simulink model "optical_path"  (R2016a)
settings: Solver=FixedStepDiscrete  StartTime=0.0  StopTime=250  FixedStep=0.1  RelTol=1e-3
undefined symbols (not defined in the file or in its folder): K, R
libraries: CEO x3
settings Model: Creator=rconan  LastModifiedBy=rconan
settings DataIOCC: LimitDataPoints=on  SaveFormat=Array
settings HardwareCC: ProdBitPerPointer=32  ProdLargestAtomicFloat=None  ProdIntDivRoundTo=Undefined  ProdEndianess=Unspecified  ProdWordSize=32  ProdHWDeviceType=32-bit Generic
settings ModelReferenceCC: PropagateSignalLabelsOutOfModel=off
settings ConfigComp: CovModelRefEnable=Off

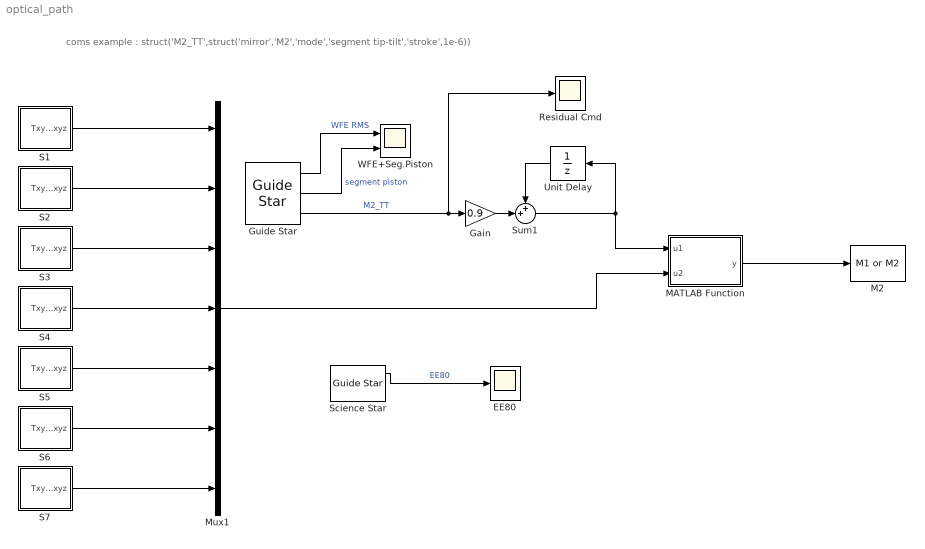
== system optical_path ==
  note: coms example : struct('M2_TT',struct('mirror','M2','mode','segment tip-tilt','stroke',1e-6))
  EE80 : Scope
  Gain : Gain  Gain=0.9
  Guide Star : CEO/Guide Star  zenith=0  azimuth=0  photometry=R - 0.640  magnitude=0  rays_origin=[0,0,25]  rays_box_size=25.5  rays_box_sampling=8  sensor=GeometricShackHartmann  n_lenslet=30  d=1  n_cam=128  px_scale=0.066  intensity_threshold=0.5  a=1  b=1  wfe_rms=on  piston=off  segment_piston=on  ee80=off  sens=off  calibration_file=[gcs,'_calibration']  coms=struct('M2_TT',struct('mirror','M2','mode','segment tip-tilt','stroke',1e-6))  coms_size=14  svd_truncation=0
  M2 : CEO/M1 or M2  mirror=M2  TxyzRxyz=on  mode_coefs=off  n_mode=66
  MATLAB Function : MATLAB Function  TreatAsAtomicUnit=on
  Mux1 : Mux  Inputs=7
  Residual Cmd : Scope
  S1 : Subsystem
  S2 : Subsystem
  S3 : Subsystem
  S4 : Subsystem
  S5 : Subsystem
  S6 : Subsystem
  S7 : Subsystem
  Science Star : CEO/Guide Star  zenith=0  azimuth=0  photometry=K - 2.179  magnitude=0  rays_origin=[0,0,25]  rays_box_size=25.5  rays_box_sampling=100  sensor=Imaging  n_lenslet=1  d=26  n_cam=128  px_scale=0.00432  intensity_threshold=0.5  a=2  b=1  wfe_rms=off  piston=off  segment_piston=off  ee80=on  sens=off  calibration_file=[]  coms=[]  coms_size=0  svd_truncation=0
  Sum1 : Sum  Inputs=++|
  Unit Delay : UnitDelay  SampleTime=-1
  WFE+Seg.Piston : Scope  NumInputPorts=2
  wires:
  Guide Star/1 -> WFE+Seg.Piston/1  "WFE RMS"
  Guide Star/2 -> WFE+Seg.Piston/2  "segment piston"
  Gain/1 -> Sum1/2
  Sum1/1 -> MATLAB Function/1(u1), Unit Delay/1
  Unit Delay/1 -> Sum1/1
  Mux1/1 -> MATLAB Function/2(u2)
  S7/1(TxyzRxyz) -> Mux1/7
  S6/1(TxyzRxyz) -> Mux1/6
  S5/1(TxyzRxyz) -> Mux1/5
  S4/1(TxyzRxyz) -> Mux1/4
  S3/1(TxyzRxyz) -> Mux1/3
  S2/1(TxyzRxyz) -> Mux1/2
  S1/1(TxyzRxyz) -> Mux1/1
  MATLAB Function/1(y) -> M2/1
  Guide Star/3 -> Gain/1, Residual Cmd/1  "M2_TT"
  Science Star/1 -> EE80/1  "EE80"

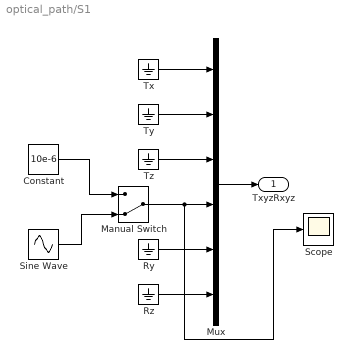
== system optical_path/S1 ==
  Constant : Constant  Value=10e-6
  Manual Switch : ManualSwitch  CurrentSetting=0
  Mux : Mux  Inputs=6
  Ry : Ground
  Rz : Ground
  Scope : Scope
  Sine Wave : Sin  SineType=Sample based  Amplitude=10e-6  Samples=100  SampleTime=1
  Tx : Ground
  Ty : Ground
  Tz : Ground
  TxyzRxyz : Outport  OutDataTypeStr=double
  wires:
  Ty/1 -> Mux/2
  Tz/1 -> Mux/3
  Ry/1 -> Mux/5
  Mux/1 -> TxyzRxyz/1
  Rz/1 -> Mux/6
  Tx/1 -> Mux/1
  Manual Switch/1 -> Scope/1, Mux/4
  Constant/1 -> Manual Switch/1
  Sine Wave/1 -> Manual Switch/2

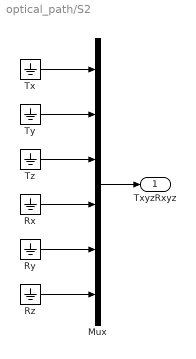
== system optical_path/S2 ==
  Mux : Mux  Inputs=6
  Rx : Ground
  Ry : Ground
  Rz : Ground
  Tx : Ground
  Ty : Ground
  Tz : Ground
  TxyzRxyz : Outport  OutDataTypeStr=double
  wires:
  Tx/1 -> Mux/1
  Ty/1 -> Mux/2
  Tz/1 -> Mux/3
  Rx/1 -> Mux/4
  Ry/1 -> Mux/5
  Mux/1 -> TxyzRxyz/1
  Rz/1 -> Mux/6

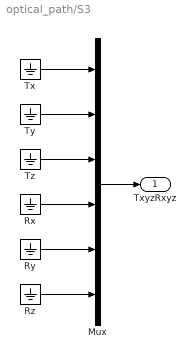
== system optical_path/S3 ==
  Mux : Mux  Inputs=6
  Rx : Ground
  Ry : Ground
  Rz : Ground
  Tx : Ground
  Ty : Ground
  Tz : Ground
  TxyzRxyz : Outport  OutDataTypeStr=double
  wires:
  Tx/1 -> Mux/1
  Ty/1 -> Mux/2
  Tz/1 -> Mux/3
  Rx/1 -> Mux/4
  Ry/1 -> Mux/5
  Mux/1 -> TxyzRxyz/1
  Rz/1 -> Mux/6

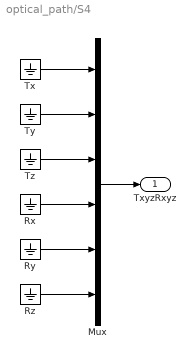
== system optical_path/S4 ==
  Mux : Mux  Inputs=6
  Rx : Ground
  Ry : Ground
  Rz : Ground
  Tx : Ground
  Ty : Ground
  Tz : Ground
  TxyzRxyz : Outport  OutDataTypeStr=double
  wires:
  Tx/1 -> Mux/1
  Ty/1 -> Mux/2
  Tz/1 -> Mux/3
  Rx/1 -> Mux/4
  Ry/1 -> Mux/5
  Mux/1 -> TxyzRxyz/1
  Rz/1 -> Mux/6

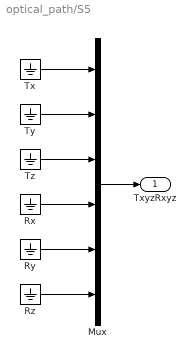
== system optical_path/S5 ==
  Mux : Mux  Inputs=6
  Rx : Ground
  Ry : Ground
  Rz : Ground
  Tx : Ground
  Ty : Ground
  Tz : Ground
  TxyzRxyz : Outport  OutDataTypeStr=double
  wires:
  Tx/1 -> Mux/1
  Ty/1 -> Mux/2
  Tz/1 -> Mux/3
  Rx/1 -> Mux/4
  Ry/1 -> Mux/5
  Mux/1 -> TxyzRxyz/1
  Rz/1 -> Mux/6

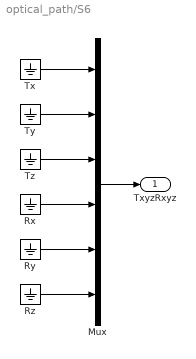
== system optical_path/S6 ==
  Mux : Mux  Inputs=6
  Rx : Ground
  Ry : Ground
  Rz : Ground
  Tx : Ground
  Ty : Ground
  Tz : Ground
  TxyzRxyz : Outport  OutDataTypeStr=double
  wires:
  Tx/1 -> Mux/1
  Ty/1 -> Mux/2
  Rx/1 -> Mux/4
  Ry/1 -> Mux/5
  Mux/1 -> TxyzRxyz/1
  Rz/1 -> Mux/6
  Tz/1 -> Mux/3

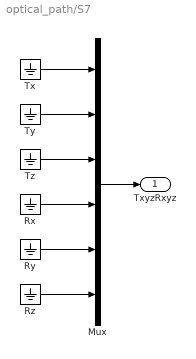
== system optical_path/S7 ==
  Mux : Mux  Inputs=6
  Rx : Ground
  Ry : Ground
  Rz : Ground
  Tx : Ground
  Ty : Ground
  Tz : Ground
  TxyzRxyz : Outport  OutDataTypeStr=double
  wires:
  Tx/1 -> Mux/1
  Ty/1 -> Mux/2
  Tz/1 -> Mux/3
  Rx/1 -> Mux/4
  Ry/1 -> Mux/5
  Mux/1 -> TxyzRxyz/1
  Rz/1 -> Mux/6

== matlab function optical_path/MATLAB Function ==
  data: u1 input; y output; u2 input
function y = diff(u1,u2)
%#codegen

u2 = reshape(u2,6,7);
u1 = reshape(u1,2,7);
u2(4:5,:) = u2(4:5,:) - u1;
y = u2';
